simulink model "axi_qpsk_rx_dec"  (R2017b)
settings: Solver=VariableStepAuto  StartTime=0.0  StopTime=10.0  RelTol=1e-3
PreLoadFcn:
  | design_filters_rx;      % run script to generate filter designs.
  | 
  | Rb = 10000;   % 1kbit / s
  | 
  | Rsym = Rb/2;   % 2 bits per symbol
  | 
  | Rsymbol = Rb/2;
  | 
  | OSR = 32;
  | 
  | f_error = 120;
  | 
  | fc = 100e3;
InitFcn:
  | fs_in=25.6e6;
values from neighbouring files (symbols this model uses):
  R_CIC = 320    [design_filters_rx.m]
  R_CICcomp = 2    [design_filters_rx.m]
  R_HB = 2    [design_filters_rx.m]
  R_RRC = 4    [design_filters_rx.m]
undefined symbols (not defined in the file or in its folder): AXI4, designMultirateFIR, Lite
libraries: xbsIndex_r4 x82, dspmlti4 x12, dsparch4 x2, dspsrcs4 x2, commrandsrc2 x1, commdigbbndpm3 x1
(part 2 of 2)

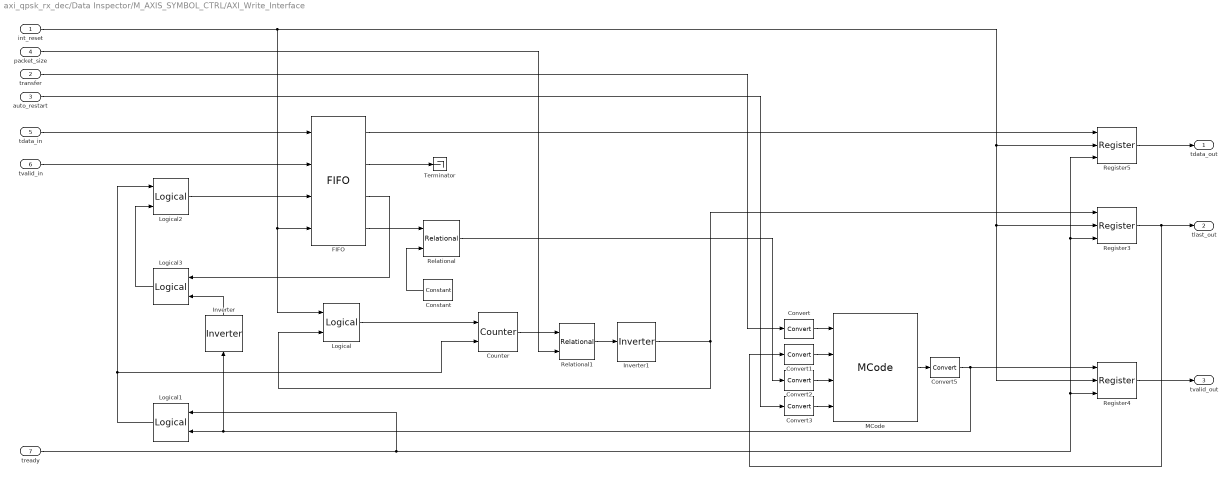
== system axi_qpsk_rx_dec/Data Inspector/M_AXIS_SYMBOL_CTRL/AXI_Write_Interface ==
  int_reset : Inport
  transfer : Inport  Port=2
  auto_restart : Inport  Port=3
  packet_size : Inport  Port=4
  tdata_in : Inport  Port=5
  tvalid_in : Inport  Port=6
  tready : Inport  Port=7
  Constant : xbsIndex_r4/Constant  const=256  gui_display_data_type=Fixed-point  arith_type=Unsigned  n_bits=11  bin_pt=0  preci_type=Single  exp_width=8  frac_width=24  explicit_period=on  period=1/fs_in  equ=P=C  opselect=C  inp2=PCIN>>17  opr=+  inp1=P  carry=CIN  dbl_ovrd=off  block_type=constant
  Convert{,1..3} (4 alike) : xbsIndex_r4/Convert  gui_display_data_type=Fixed-point  arith_type=Unsigned  n_bits=1  bin_pt=0  float_type=Single  exp_bits=8  fraction_bits=24  quantization=Truncate  overflow=Wrap  en=off  latency=0  pipeline=off  dbl_ovrd=off  block_type=convert
  Convert5 : xbsIndex_r4/Convert  gui_display_data_type=Boolean  arith_type=Boolean  n_bits=1  bin_pt=0  float_type=Single  exp_bits=8  fraction_bits=24  quantization=Truncate  overflow=Wrap  en=off  latency=0  pipeline=off  dbl_ovrd=off  block_type=convert
  Counter : xbsIndex_r4/Counter  cnt_type=Free Running  cnt_to=Inf  operation=Up  start_count=0  cnt_by_val=1  arith_type=Unsigned  n_bits=32  bin_pt=0  load_pin=off  rst=on  en=on  explicit_period=on  period=1/fs_in  use_behavioral_HDL=off  implementation=Fabric  dbl_ovrd=off  block_type=counter
  FIFO : xbsIndex_r4/FIFO  mem_type=Block RAM  performance_options=Standard_FIFO  embedded_registers=off  depth=512  percent_nbits=1  rst=on  rst_latency=2  en=off  use_dcount=on  use_percent_full_port=off  use_almost_empty=off  almost_empty_thresh=2  use_almost_full=off  almost_full_thresh=14  explicit_period=off  dbl_ovrd=off  block_type=fifo
  Inverter : xbsIndex_r4/Inverter  en=off  latency=0  dbl_ovrd=off  block_type=inv
  Inverter1 : xbsIndex_r4/Inverter  en=off  latency=0  dbl_ovrd=off  block_type=inv
  Logical : xbsIndex_r4/Logical  logical_function=OR  inputs=2  en=off  latency=0  precision=Full  arith_type=Unsigned  n_bits=16  bin_pt=0  align_bp=on  dbl_ovrd=off  block_type=logical
  Logical1 : xbsIndex_r4/Logical  logical_function=AND  inputs=2  en=off  latency=0  precision=Full  arith_type=Unsigned  n_bits=16  bin_pt=0  align_bp=on  dbl_ovrd=off  block_type=logical
  Logical2 : xbsIndex_r4/Logical  logical_function=OR  inputs=2  en=off  latency=0  precision=Full  arith_type=Unsigned  n_bits=16  bin_pt=0  align_bp=on  dbl_ovrd=off  block_type=logical
  Logical3 : xbsIndex_r4/Logical  logical_function=AND  inputs=2  en=off  latency=0  precision=Full  arith_type=Unsigned  n_bits=16  bin_pt=0  align_bp=on  dbl_ovrd=off  block_type=logical
  MCode : xbsIndex_r4/MCode  mfname=CtrlFSM  explicit_period=on  period=1/fs_in  inputsTable={'boundInpExpr'=>['','','',''],'inputs'=>['AXIwrite','tlast','dcount','AXIauto']}  outputsTable={'outputs'=>['re'],'suppressOut'=>['off']}  enable_stdout=off  enable_debug=off  suppress_output=on  defparams={}  hide_port_list={}  dbl_ovrd=off  block_type=mcode
  Register3 : xbsIndex_r4/Register  init=0  rst=on  en=on  dbl_ovrd=off  block_type=register
  Register4 : xbsIndex_r4/Register  init=0  rst=on  en=on  dbl_ovrd=off  block_type=register
  Register5 : xbsIndex_r4/Register  init=0  rst=on  en=on  dbl_ovrd=off  block_type=register
  Relational : xbsIndex_r4/Relational  mode=a>=b  op_type=Bool  en=off  latency=0  dbl_ovrd=off  block_type=relational
  Relational1 : xbsIndex_r4/Relational  mode=a<b  op_type=Bool  en=off  latency=0  dbl_ovrd=off  block_type=relational
  Terminator : Terminator
  tdata_out : Outport
  tlast_out : Outport  Port=2
  tvalid_out : Outport  Port=3
  wires:
  Register5/1 -> tdata_out/1
  FIFO/2 -> Terminator/1
  Logical2/1 -> FIFO/3
  Convert1/1 -> MCode/2
  Convert/1 -> MCode/1
  transfer/1 -> Convert/1
  int_reset/1 -> Logical/1, FIFO/4, Register5/2, Register3/2, Register4/2
  Inverter/1 -> Logical3/2
  tready/1 -> Register3/3, Register5/3, Register4/3, Logical1/1
  Convert3/1 -> MCode/4
  Convert2/1 -> MCode/3
  Inverter1/1 -> Logical/2, Register3/1
  Logical1/1 -> Logical2/1, Counter/2
  tdata_in/1 -> FIFO/1
  FIFO/3 -> Logical3/1
  Relational1/1 -> Inverter1/1
  Counter/1 -> Relational1/1
  Logical/1 -> Counter/1
  Relational/1 -> Convert2/1
  Constant/1 -> Relational/2
  packet_size/1 -> Relational1/2
  MCode/1 -> Convert5/1
  Logical3/1 -> Logical2/2
  auto_restart/1 -> Convert3/1
  FIFO/4 -> Relational/1
  Register3/1 -> Convert1/1, tlast_out/1
  Register4/1 -> tvalid_out/1
  Convert5/1 -> Register4/1, Inverter/1, Logical1/2
  FIFO/1 -> Register5/1
  tvalid_in/1 -> FIFO/2
